simulink model "examples"  (R2016a)
settings: Solver=VariableStepAuto  StartTime=0.0  StopTime=10.0  RelTol=1e-3
settings Model: Creator=KamalEldeen  LastModifiedBy=KamalEldeen

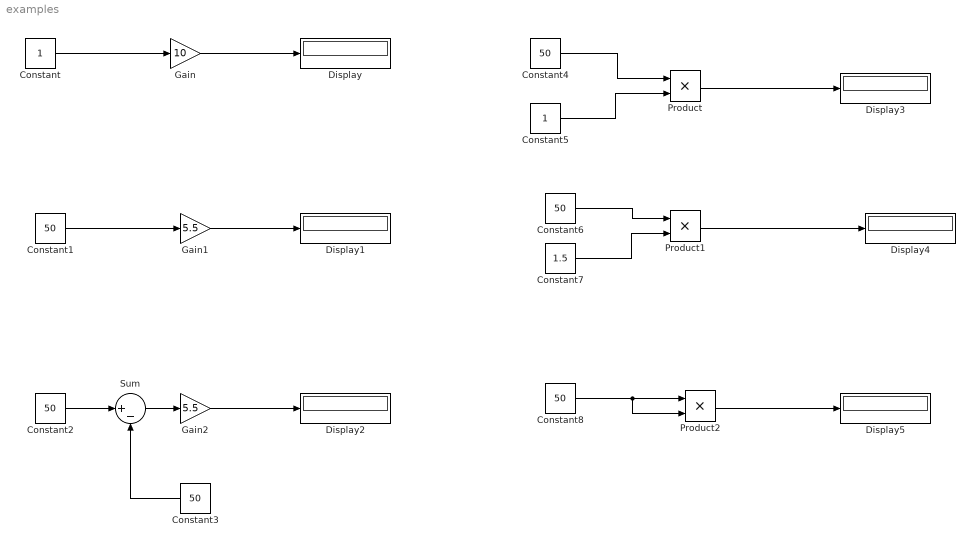
== system examples ==
  Constant : Constant
  Constant{1..4,6,8} (6 alike) : Constant  Value=50
  Constant5 : Constant
  Constant7 : Constant  Value=1.5
  Display{,1..5} (6 alike) : Display
  Gain : Gain  Gain=10
  Gain1 : Gain  Gain=5.5
  Gain2 : Gain  Gain=5.5
  Product : Product
  Product1 : Product
  Product2 : Product
  Sum : Sum  Inputs=|+-
  wires:
  Constant/1 -> Gain/1
  Gain/1 -> Display/1
  Constant1/1 -> Gain1/1
  Gain1/1 -> Display1/1
  Gain2/1 -> Display2/1
  Constant2/1 -> Sum/1
  Sum/1 -> Gain2/1
  Constant3/1 -> Sum/2
  Constant4/1 -> Product/1
  Constant5/1 -> Product/2
  Constant6/1 -> Product1/1
  Constant7/1 -> Product1/2
  Constant8/1 -> Product2/2, Product2/1
  Product2/1 -> Display5/1
  Product1/1 -> Display4/1
  Product/1 -> Display3/1
